simulink model "Train_local_R2021a"  (R2021a)
settings: Solver=FixedStepAuto  StartTime=0.0  StopTime=Inf  FixedStep=1/1000  RelTol=1e-3  EnableMultiTasking=on
libraries: rllib x1
settings Model: Creator=Ammar  LastModifiedBy=vic-b
settings SolverCC: AlgebraicLoopSolver=TrustRegion  PositivePriorityOrder=on  AutoInsertRateTranBlk=on
settings OptimizationCC: EnhancedBackFolding=on  PassReuseOutputArgsThreshold=0  MaxStackSize=64  OptimizeBlockOrder=speed  DifferentSizesBufferReuse=on  OptimizationCustomize=off
settings DebuggingCC: ParameterTunabilityLossMsg=error  SFMachineParentedDataDiag=warning  ArithmeticOperatorsInVariantConditions=warning
settings HardwareCC: ProdBitPerPointer=32  ProdBitPerSizeT=32  ProdBitPerPtrDiffT=32  ProdLargestAtomicInteger=Long  ProdLargestAtomicFloat=Double  ProdWordSize=32  ProdHWDeviceType=ARM Compatible->ARM Cortex  UseEmbeddedCoderFeatures=off  UseSimulinkCoderFeatures=off
settings SFSimCC: SimUseLocalCustomCode=off  MATLABDynamicMemAlloc=off  CustomCodeUndefinedFunction=UseInterfaceOnly  SimTargetLang=C++
settings RTWCC: SystemTargetFile=ert.tlc  HardwareBoard=Raspberry Pi  TLCOptions="-aInlineSetEventsForThisBaseRateFcn=TLC_FALSE -aSuppressMultiTaskScheduler=TLC_FALSE  -aRateBasedStepFcn=0"  TemplateMakefile=ert_default_tmf  GenerateReport=on  RTWUseLocalCustomCode=off  Toolchain=GNU GCC Embedded Linux  BuildConfiguration=Faster Runs  LaunchReport=on
settings CodeAppCC: ForceParamTrailComments=on  OperatorAnnotations=on
settings ERTTargetCC: ERTCustomFileBanners=off  SupportContinuousTime=on  SupportNonInlinedSFcns=on  RemoveResetFunc=off  SupportVariableSizeSignals=on  ModelStepFunctionPrototypeControlCompliant=off

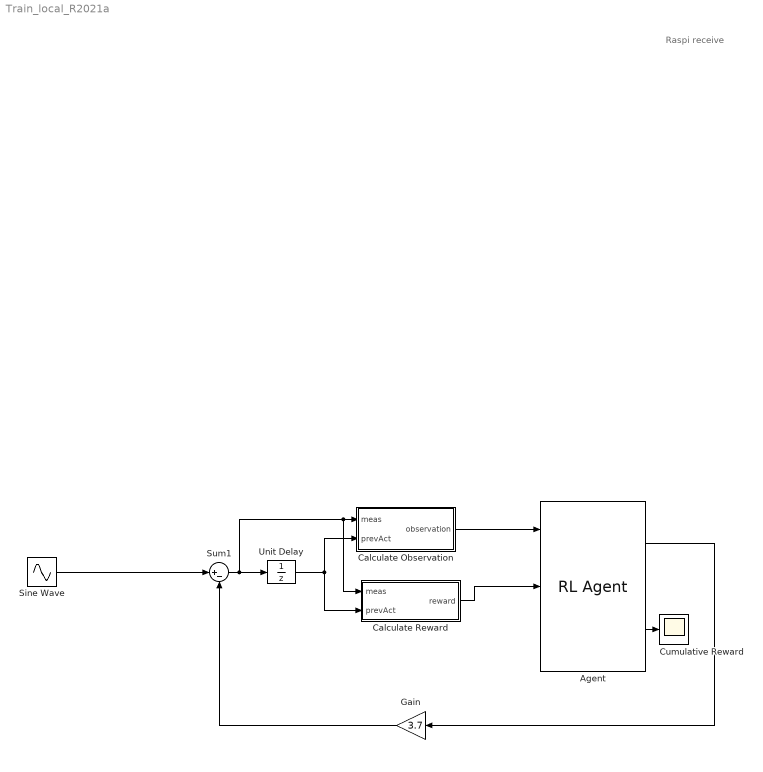
== system Train_local_R2021a ==
  note: Raspi receive
  Agent : rllib/RL Agent  Agent=agent  ExternalActionAsInput=off  ProvideCumRwd=on  TreatAsDirectFeedthrough=on
      settings: SourceProductName=Reinforcement Learning
  Calculate Observation : Subsystem
  Calculate Reward : Subsystem
  Cumulative Reward : Scope
  Gain : Gain  Gain=3.7
  Sine Wave : Sin  SampleTime=0
  Sum1 : Sum  Inputs=|+-
  Unit Delay : UnitDelay  SampleTime=-1  HasFrameUpgradeWarning=on
  wires:
  Sine Wave/1 -> Sum1/1
  Sum1/1 -> Calculate Reward/1(meas), Calculate Observation/1(meas), Unit Delay/1
  Calculate Observation/1(observation) -> Agent/1
  Unit Delay/1 -> Calculate Observation/2(prevAct), Calculate Reward/2(prevAct)
  Agent/2 -> Cumulative Reward/1
  Gain/1 -> Sum1/2
  Agent/1 -> Gain/1
  Calculate Reward/1(reward) -> Agent/2

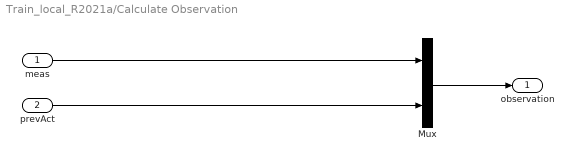
== system Train_local_R2021a/Calculate Observation ==
  meas : Inport
  prevAct : Inport  Port=2
  Mux : Mux  Inputs=2
  observation : Outport  VectorParamsAs1DForOutWhenUnconnected=off
  wires:
  Mux/1 -> observation/1
  meas/1 -> Mux/1
  prevAct/1 -> Mux/2

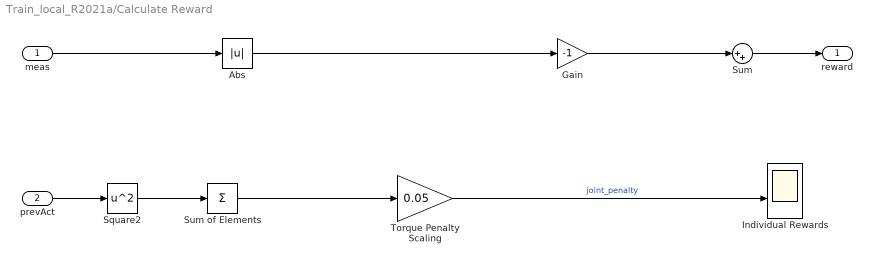
== system Train_local_R2021a/Calculate Reward ==
  meas : Inport
  prevAct : Inport  Port=2
  Abs : Abs
  Gain : Gain  Gain=-1
  Individual Rewards : Scope  NumInputPorts=4
  Square2 : Math  Operator=square  SignedPower=on  SaturateOnIntegerOverflow=on
  Sum : Sum  Inputs=|++
  Sum of Elements : Sum  Inputs=+
  Torque Penalty Scaling : Gain  Gain=0.05
  reward : Outport  VectorParamsAs1DForOutWhenUnconnected=off
  wires:
  meas/1 -> Abs/1
  Sum of Elements/1 -> Torque Penalty Scaling/1
  prevAct/1 -> Square2/1
  Square2/1 -> Sum of Elements/1
  Torque Penalty Scaling/1 -> Individual Rewards/3  "joint_penalty"
  Abs/1 -> Gain/1
  Gain/1 -> Sum/1
  Sum/1 -> reward/1
